simulink model "RateGyro_to_EulerAngles"  (R2020b)
settings: Solver=VariableStepAuto  StartTime=0.0  StopTime=50.0  RelTol=1e-3
settings Model: Creator=dariusmensah  LastModifiedBy=dariusmensah

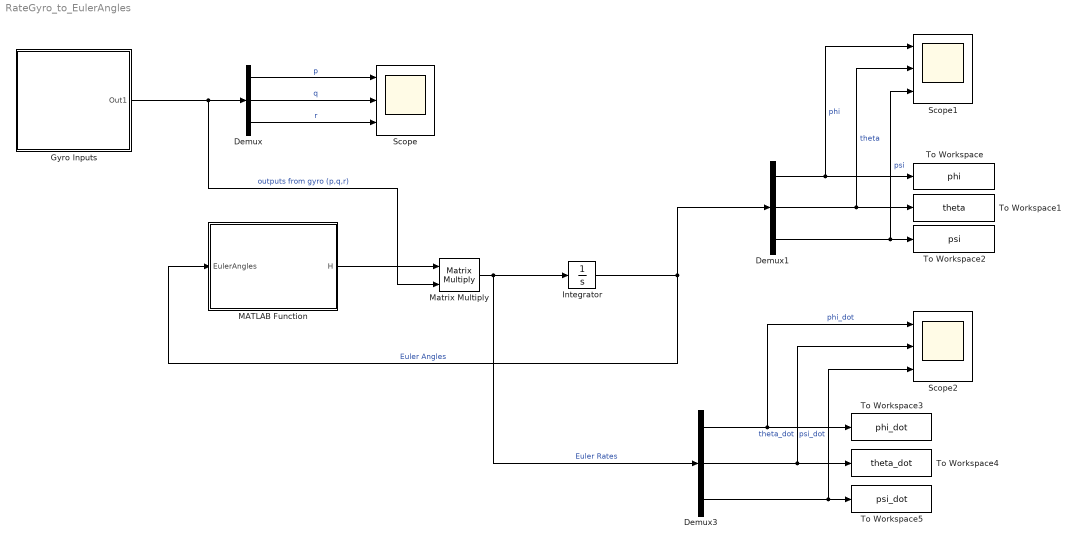
== system RateGyro_to_EulerAngles ==
  Demux : Demux  Outputs=3
  Demux1 : Demux  Outputs=3
  Demux3 : Demux  Outputs=3
  Gyro Inputs : Subsystem
  Integrator : Integrator  InitialCondition=[0;0;0]
  MATLAB Function : MATLAB Function  TreatAsAtomicUnit=on
  Matrix Multiply : Product  Multiplication=Matrix(*)
  Scope : Scope  NumInputPorts=3
  Scope1 : Scope  NumInputPorts=3
  Scope2 : Scope  NumInputPorts=3
  To Workspace : ToWorkspace  VariableName=phi  SaveFormat=Structure With Time  SampleTime=-1
  To Workspace1 : ToWorkspace  VariableName=theta  SaveFormat=Structure With Time  SampleTime=-1
  To Workspace2 : ToWorkspace  VariableName=psi  SaveFormat=Structure With Time  SampleTime=-1
  To Workspace3 : ToWorkspace  VariableName=phi_dot  SaveFormat=Structure With Time  SampleTime=-1
  To Workspace4 : ToWorkspace  VariableName=theta_dot  SaveFormat=Structure With Time  SampleTime=-1
  To Workspace5 : ToWorkspace  VariableName=psi_dot  SaveFormat=Structure With Time  SampleTime=-1
  wires:
  Gyro Inputs/1(Out1) -> Matrix Multiply/2, Demux/1  "outputs from gyro (p,q,r)"
  Demux/1 -> Scope/1  "p"
  Demux/2 -> Scope/2  "q"
  Demux/3 -> Scope/3  "r"
  MATLAB Function/1(H) -> Matrix Multiply/1
  Matrix Multiply/1 -> Demux3/1, Integrator/1  "Euler Rates"
  Integrator/1 -> Demux1/1, MATLAB Function/1(EulerAngles)  "Euler Angles"
  Demux1/1 -> To Workspace/1, Scope1/1  "phi"
  Demux1/2 -> To Workspace1/1, Scope1/2  "theta"
  Demux1/3 -> Scope1/3, To Workspace2/1  "psi"
  Demux3/1 -> To Workspace3/1, Scope2/1  "phi_dot"
  Demux3/2 -> To Workspace4/1, Scope2/2  "theta_dot"
  Demux3/3 -> Scope2/3, To Workspace5/1  "psi_dot"

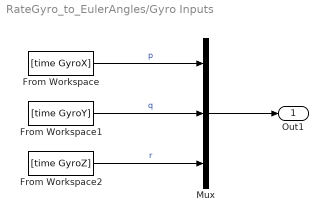
== system RateGyro_to_EulerAngles/Gyro Inputs ==
  From Workspace : FromWorkspace  VariableName=[time GyroX]
  From Workspace1 : FromWorkspace  VariableName=[time GyroY]
  From Workspace2 : FromWorkspace  VariableName=[time GyroZ]
  Mux : Mux  Inputs=3
  Out1 : Outport
  wires:
  From Workspace2/1 -> Mux/3  "r"
  From Workspace/1 -> Mux/1  "p"
  From Workspace1/1 -> Mux/2  "q"
  Mux/1 -> Out1/1

== matlab function RateGyro_to_EulerAngles/MATLAB Function ==
  data: EulerAngles input; H output
function H = EulerKinematicEq (EulerAngles)

phi = EulerAngles(1);
theta = EulerAngles(2);


H = [1 -sind(phi)*tand(theta) cosd(phi)*tand(theta); 
       0 cosd(phi) sind(phi);
       0 -sind(phi)*secd(theta) cosd(phi)*secd(theta)];
end
